simulink model "lektion8"  (R2024a)
settings: Solver=VariableStepAuto  StartTime=0.0  StopTime=10.0  RelTol=1e-3
undefined symbols (not defined in the file or in its folder): T
settings Model: Creator=jacob  LastModifiedBy=jacob

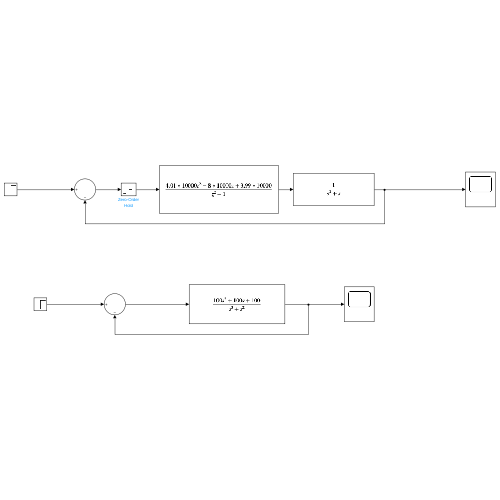
[thumbnail: Simulink's stored preview of the top-level diagram]
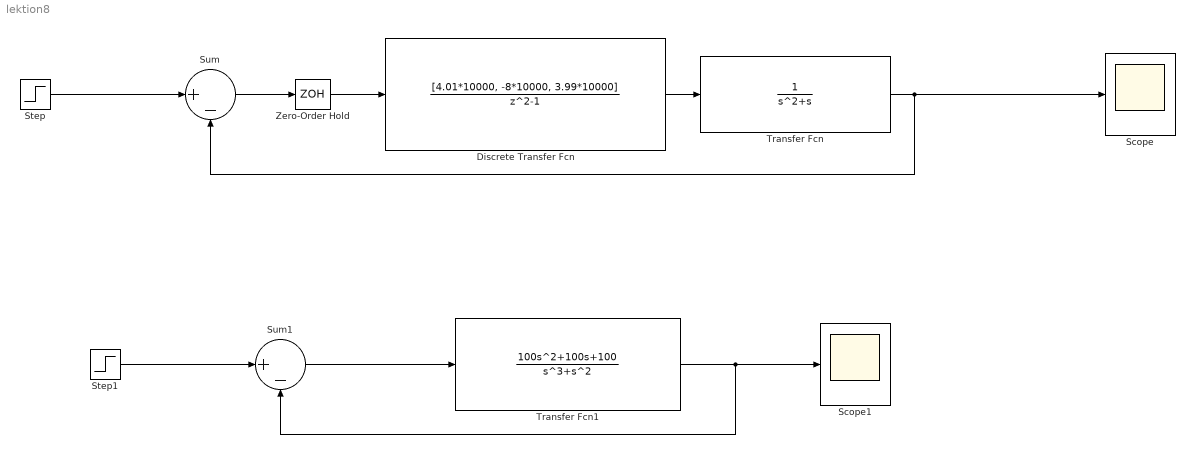
== system lektion8 ==
  Discrete Transfer Fcn : DiscreteTransferFcn  Numerator=[4.01*10000, -8*10000, 3.99*10000]  Denominator=[1, 0, -1]
  Scope : Scope
  Scope1 : Scope
  Step : Step  SampleTime=0
  Step1 : Step  SampleTime=0
  Sum : Sum  Inputs=|+-
  Sum1 : Sum  Inputs=|+-
  Transfer Fcn : TransferFcn  Denominator=[1 1 0]
  Transfer Fcn1 : TransferFcn  Numerator=[100 100 100]  Denominator=[1 1 0 0]
  Zero-Order Hold : ZeroOrderHold  SampleTime=T
  wires:
  Transfer Fcn/1 -> Sum/2, Scope/1
  Sum/1 -> Zero-Order Hold/1
  Step/1 -> Sum/1
  Transfer Fcn1/1 -> Sum1/2, Scope1/1
  Step1/1 -> Sum1/1
  Sum1/1 -> Transfer Fcn1/1
  Discrete Transfer Fcn/1 -> Transfer Fcn/1
  Zero-Order Hold/1 -> Discrete Transfer Fcn/1
